simulink subsystem "DCDC_Converters_GenBat"  (R2024a)
settings: Solver=VariableStepAuto  StartTime=0.0  StopTime=10.0  RelTol=1e-3
undefined symbols (not defined in the file): C_bus, DCDC, L_boost, R_boost, rPre
settings Model: Creator=Henrique Mesquita  LastModifiedBy=henri

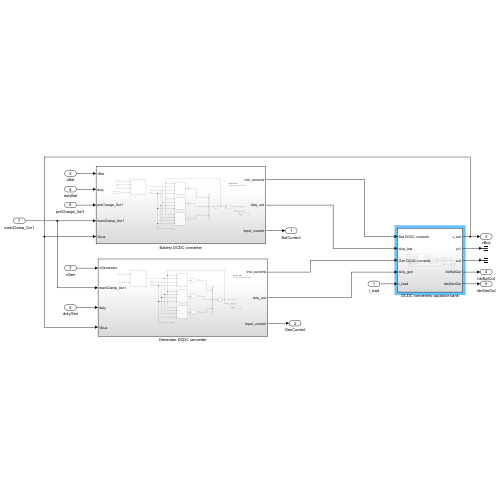
[thumbnail: Simulink's stored preview of the top-level diagram]
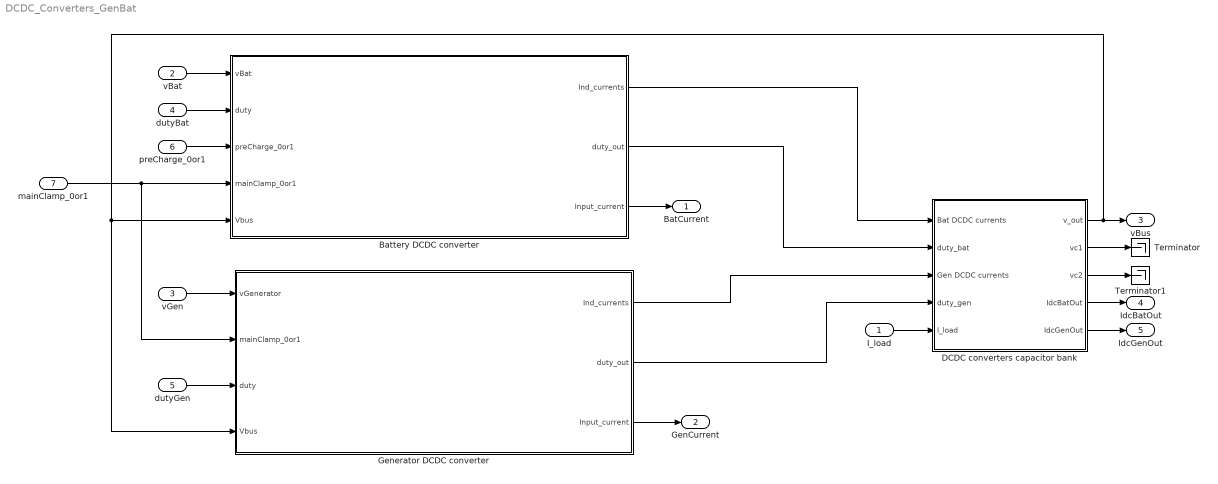
== system DCDC_Converters_GenBat ==
  I_load : Inport
  vBat : Inport  Port=2
  vGen : Inport  Port=3
  dutyBat : Inport  Port=4
  dutyGen : Inport  Port=5
  preCharge_0or1 : Inport  Port=6  OutDataTypeStr=int8
  mainClamp_0or1 : Inport  Port=7  OutDataTypeStr=int8
  Battery DCDC converter : Subsystem
  DCDC converters capacitor bank : Subsystem
  Generator DCDC converter : Subsystem
  Terminator : Terminator
  Terminator1 : Terminator
  BatCurrent : Outport
  GenCurrent : Outport  Port=2
  vBus : Outport  Port=3
  IdcBatOut : Outport  Port=4
  IdcGenOut : Outport  Port=5
  wires:
  Battery DCDC converter/1(Ind_currents) -> DCDC converters capacitor bank/1(Bat DCDC currents)
  Generator DCDC converter/1(Ind_currents) -> DCDC converters capacitor bank/3(Gen DCDC currents)
  Battery DCDC converter/2(duty_out) -> DCDC converters capacitor bank/2(duty_bat)
  Generator DCDC converter/2(duty_out) -> DCDC converters capacitor bank/4(duty_gen)
  I_load/1 -> DCDC converters capacitor bank/5(I_load)
  Battery DCDC converter/3(Input_current) -> BatCurrent/1
  Generator DCDC converter/3(Input_current) -> GenCurrent/1
  vGen/1 -> Generator DCDC converter/1(vGenerator)
  dutyGen/1 -> Generator DCDC converter/3(duty)
  preCharge_0or1/1 -> Battery DCDC converter/3(preCharge_0or1)
  mainClamp_0or1/1 -> Generator DCDC converter/2(mainClamp_0or1), Battery DCDC converter/4(mainClamp_0or1)
  dutyBat/1 -> Battery DCDC converter/2(duty)
  vBat/1 -> Battery DCDC converter/1(vBat)
  DCDC converters capacitor bank/1(v_out) -> vBus/1, Generator DCDC converter/4(Vbus), Battery DCDC converter/5(Vbus)
  DCDC converters capacitor bank/2(vc1) -> Terminator/1
  DCDC converters capacitor bank/3(vc2) -> Terminator1/1
  DCDC converters capacitor bank/4(IdcBatOut) -> IdcBatOut/1
  DCDC converters capacitor bank/5(IdcGenOut) -> IdcGenOut/1

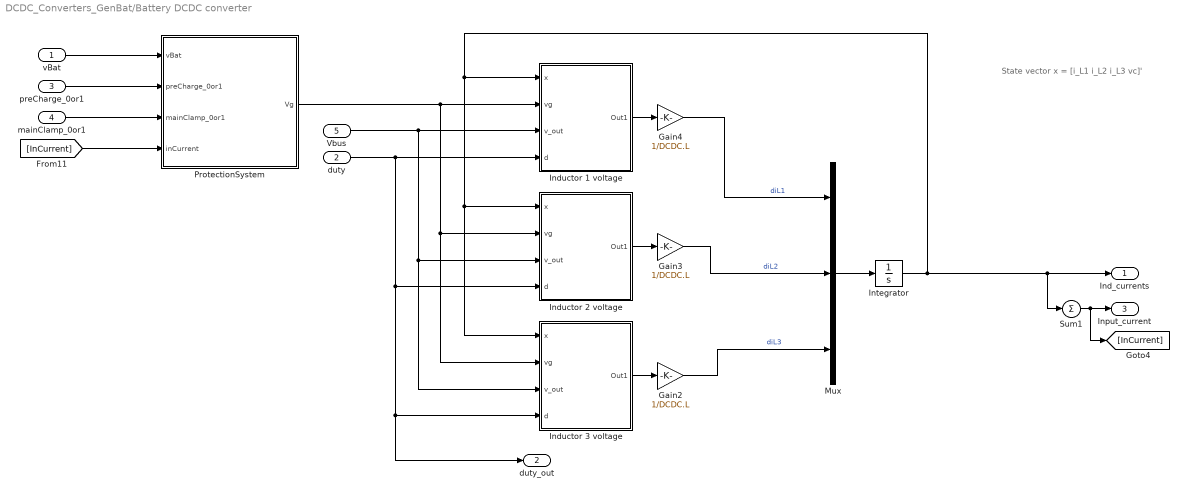
== system DCDC_Converters_GenBat/Battery DCDC converter ==
  note: State vector
      | x = [i_L1 i_L2 i_L3 vc]'
  vBat : Inport
  duty : Inport  Port=2
  preCharge_0or1 : Inport  Port=3
  mainClamp_0or1 : Inport  Port=4
  Vbus : Inport  Port=5
  Gain2 : Gain  Gain=1/DCDC.L
  Gain3 : Gain  Gain=1/DCDC.L
  Gain4 : Gain  Gain=1/DCDC.L
  Inductor 1 voltage : Subsystem
  Inductor 2 voltage : Subsystem
  Inductor 3 voltage : Subsystem
  Integrator : Integrator  InitialCondition=[0;0;0]
  Mux : Mux  Inputs=3
  ProtectionSystem : Subsystem
  Sum1 : Sum  Inputs=+
  Ind_currents : Outport
  duty_out : Outport  Port=2
  Input_current : Outport  Port=3
  wires:
  [InCurrent] -> ProtectionSystem/4(inCurrent)
  mainClamp_0or1/1 -> ProtectionSystem/3(mainClamp_0or1)
  preCharge_0or1/1 -> ProtectionSystem/2(preCharge_0or1)
  vBat/1 -> ProtectionSystem/1(vBat)
  Sum1/1 -> Input_current/1, [InCurrent]
  duty/1 -> duty_out/1, Inductor 3 voltage/4(d), Inductor 2 voltage/4(d), Inductor 1 voltage/4(d)
  ProtectionSystem/1(Vg) -> Inductor 2 voltage/2(vg), Inductor 3 voltage/2(vg), Inductor 1 voltage/2(vg)
  Vbus/1 -> Inductor 1 voltage/3(v_out), Inductor 3 voltage/3(v_out), Inductor 2 voltage/3(v_out)
  Integrator/1 -> Inductor 1 voltage/1(x), Inductor 3 voltage/1(x), Inductor 2 voltage/1(x), Ind_currents/1, Sum1/1
  Gain4/1 -> Mux/1  "diL1"
  Gain3/1 -> Mux/2  "diL2"
  Gain2/1 -> Mux/3  "diL3"
  Inductor 1 voltage/1(Out1) -> Gain4/1
  Inductor 3 voltage/1(Out1) -> Gain2/1
  Inductor 2 voltage/1(Out1) -> Gain3/1
  Mux/1 -> Integrator/1

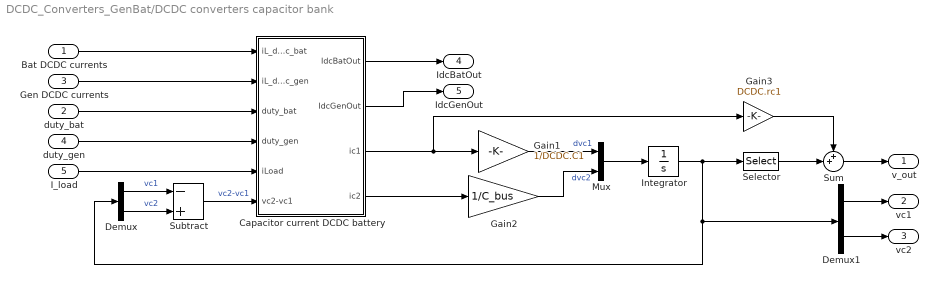
== system DCDC_Converters_GenBat/DCDC converters capacitor bank ==
  Bat DCDC currents : Inport
  duty_bat : Inport  Port=2
  Gen DCDC currents : Inport  Port=3
  duty_gen : Inport  Port=4
  I_load : Inport  Port=5
  Capacitor current DCDC battery : Subsystem
  Demux : Demux  Outputs=2
  Demux1 : Demux  Outputs=2
  Gain1 : Gain  Gain=1/DCDC.C1
  Gain2 : Gain  Gain=1/C_bus
  Gain3 : Gain  Gain=DCDC.rc1
  Integrator : Integrator
  Mux : Mux  Inputs=2
  Selector : Selector  InputPortWidth=2  IndexOptions=Index vector (dialog)  Indices=[1]  OutputSizes=1
  Subtract : Sum  Inputs=-+
  Sum : Sum  Inputs=++|
  v_out : Outport
  vc1 : Outport  Port=2
  vc2 : Outport  Port=3
  IdcBatOut : Outport  Port=4
  IdcGenOut : Outport  Port=5
  wires:
  Mux/1 -> Integrator/1
  Demux/1 -> Subtract/1  "vc1"
  Demux/2 -> Subtract/2  "vc2"
  Bat DCDC currents/1 -> Capacitor current DCDC battery/1(iL_dcdc_bat)
  Gen DCDC currents/1 -> Capacitor current DCDC battery/2(iL_dcdc_gen)
  I_load/1 -> Capacitor current DCDC battery/5(iLoad)
  Subtract/1 -> Capacitor current DCDC battery/6(vc2-vc1)  "vc2-vc1"
  Capacitor current DCDC battery/4(ic2) -> Gain2/1
  Capacitor current DCDC battery/3(ic1) -> Gain3/1, Gain1/1
  Gain1/1 -> Mux/1  "dvc1"
  Gain2/1 -> Mux/2  "dvc2"
  duty_bat/1 -> Capacitor current DCDC battery/3(duty_bat)
  duty_gen/1 -> Capacitor current DCDC battery/4(duty_gen)
  Integrator/1 -> Selector/1, Demux1/1, Demux/1
  Gain3/1 -> Sum/1
  Selector/1 -> Sum/2
  Sum/1 -> v_out/1
  Demux1/1 -> vc1/1
  Demux1/2 -> vc2/1
  Capacitor current DCDC battery/1(IdcBatOut) -> IdcBatOut/1
  Capacitor current DCDC battery/2(IdcGenOut) -> IdcGenOut/1

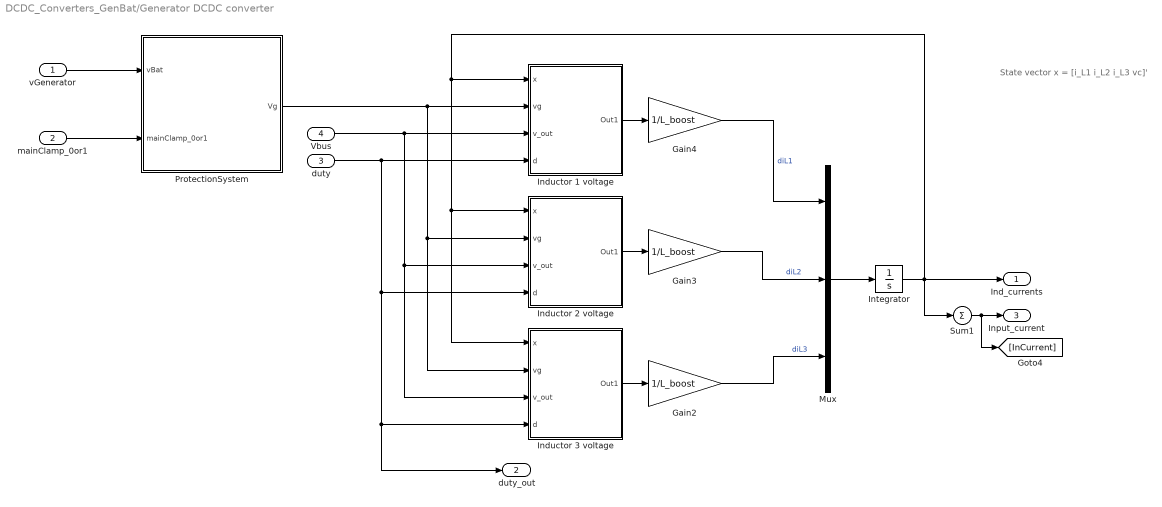
== system DCDC_Converters_GenBat/Generator DCDC converter ==
  note: State vector
      | x = [i_L1 i_L2 i_L3 vc]'
  vGenerator : Inport
  mainClamp_0or1 : Inport  Port=2
  duty : Inport  Port=3
  Vbus : Inport  Port=4
  Gain2 : Gain  Gain=1/L_boost
  Gain3 : Gain  Gain=1/L_boost
  Gain4 : Gain  Gain=1/L_boost
  Inductor 1 voltage : Subsystem
  Inductor 2 voltage : Subsystem
  Inductor 3 voltage : Subsystem
  Integrator : Integrator  InitialCondition=[0;0;0]  LimitOutput=on  LowerSaturationLimit=0
  Mux : Mux  Inputs=3
  ProtectionSystem : Subsystem
  Sum1 : Sum  Inputs=+
  Ind_currents : Outport
  duty_out : Outport  Port=2
  Input_current : Outport  Port=3
  wires:
  mainClamp_0or1/1 -> ProtectionSystem/2(mainClamp_0or1)
  vGenerator/1 -> ProtectionSystem/1(vBat)
  ProtectionSystem/1(Vg) -> Inductor 3 voltage/2(vg), Inductor 2 voltage/2(vg), Inductor 1 voltage/2(vg)
  Vbus/1 -> Inductor 1 voltage/3(v_out), Inductor 3 voltage/3(v_out), Inductor 2 voltage/3(v_out)
  duty/1 -> Inductor 2 voltage/4(d), Inductor 3 voltage/4(d), duty_out/1, Inductor 1 voltage/4(d)
  Integrator/1 -> Ind_currents/1, Sum1/1, Inductor 1 voltage/1(x), Inductor 3 voltage/1(x), Inductor 2 voltage/1(x)
  Inductor 3 voltage/1(Out1) -> Gain2/1
  Gain3/1 -> Mux/2  "diL2"
  Inductor 2 voltage/1(Out1) -> Gain3/1
  Inductor 1 voltage/1(Out1) -> Gain4/1
  Sum1/1 -> Input_current/1, [InCurrent]
  Gain4/1 -> Mux/1  "diL1"
  Mux/1 -> Integrator/1
  Gain2/1 -> Mux/3  "diL3"

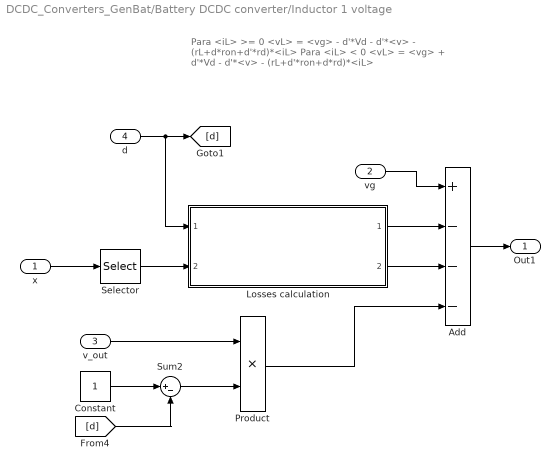
== system DCDC_Converters_GenBat/Battery DCDC converter/Inductor 1 voltage ==
  note: Para <iL> >= 0
      | <vL> = <vg> - d'*Vd - d'*<v> - (rL+d*ron+d'*rd)*<iL>
      | Para <iL> < 0
      | <vL> = <vg> + d'*Vd - d'*<v> - (rL+d'*ron+d*rd)*<iL>
  x : Inport
  vg : Inport  Port=2
  v_out : Inport  Port=3
  d : Inport  Port=4
  Add : Sum  Inputs=+---
  Constant : Constant
  Losses calculation : Subsystem  ReferencedSubsystem=Losses_calculation
  Product : Product
  Selector : Selector  InputPortWidth=3  IndexOptions=Index vector (dialog)  Indices=[1]  OutputSizes=1
  Sum2 : Sum  Inputs=|+-
  Out1 : Outport
  wires:
  Losses calculation/2 -> Add/3
  Losses calculation/1 -> Add/2
  [d] -> Sum2/2
  Sum2/1 -> Product/2
  Constant/1 -> Sum2/1
  Add/1 -> Out1/1
  Selector/1 -> Losses calculation/2
  v_out/1 -> Product/1
  d/1 -> [d], Losses calculation/1
  x/1 -> Selector/1
  Product/1 -> Add/4
  vg/1 -> Add/1

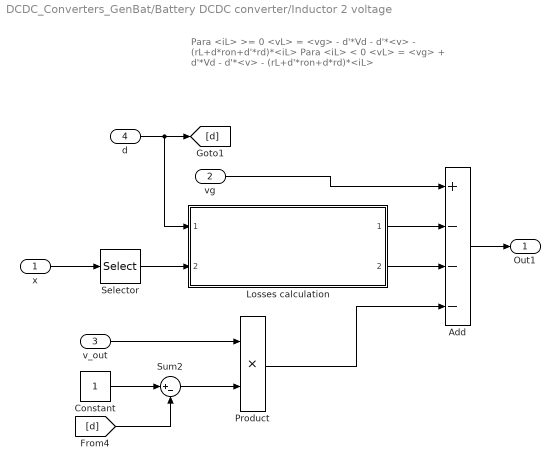
== system DCDC_Converters_GenBat/Battery DCDC converter/Inductor 2 voltage ==
  note: Para <iL> >= 0
      | <vL> = <vg> - d'*Vd - d'*<v> - (rL+d*ron+d'*rd)*<iL>
      | Para <iL> < 0
      | <vL> = <vg> + d'*Vd - d'*<v> - (rL+d'*ron+d*rd)*<iL>
  x : Inport
  vg : Inport  Port=2
  v_out : Inport  Port=3
  d : Inport  Port=4
  Add : Sum  Inputs=+---
  Constant : Constant
  Losses calculation : Subsystem  ReferencedSubsystem=Losses_calculation
  Product : Product
  Selector : Selector  InputPortWidth=3  IndexOptions=Index vector (dialog)  Indices=[2]  OutputSizes=1
  Sum2 : Sum  Inputs=|+-
  Out1 : Outport
  wires:
  Losses calculation/2 -> Add/3
  Losses calculation/1 -> Add/2
  [d] -> Sum2/2
  Sum2/1 -> Product/2
  Constant/1 -> Sum2/1
  Add/1 -> Out1/1
  Selector/1 -> Losses calculation/2
  v_out/1 -> Product/1
  d/1 -> [d], Losses calculation/1
  x/1 -> Selector/1
  Product/1 -> Add/4
  vg/1 -> Add/1

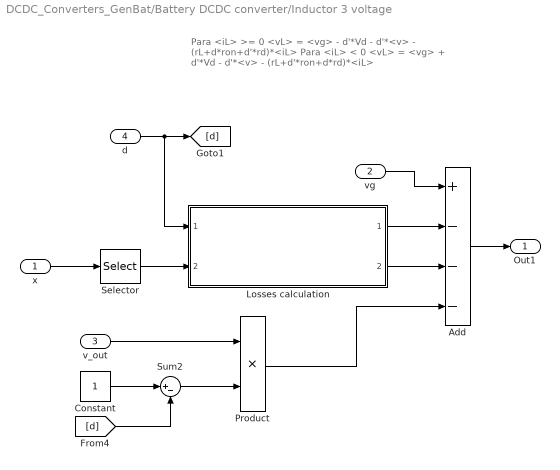
== system DCDC_Converters_GenBat/Battery DCDC converter/Inductor 3 voltage ==
  note: Para <iL> >= 0
      | <vL> = <vg> - d'*Vd - d'*<v> - (rL+d*ron+d'*rd)*<iL>
      | Para <iL> < 0
      | <vL> = <vg> + d'*Vd - d'*<v> - (rL+d'*ron+d*rd)*<iL>
  x : Inport
  vg : Inport  Port=2
  v_out : Inport  Port=3
  d : Inport  Port=4
  Add : Sum  Inputs=+---
  Constant : Constant
  Losses calculation : Subsystem  ReferencedSubsystem=Losses_calculation
  Product : Product
  Selector : Selector  InputPortWidth=3  IndexOptions=Index vector (dialog)  Indices=[3]  OutputSizes=1
  Sum2 : Sum  Inputs=|+-
  Out1 : Outport
  wires:
  Losses calculation/2 -> Add/3
  Losses calculation/1 -> Add/2
  [d] -> Sum2/2
  Sum2/1 -> Product/2
  Constant/1 -> Sum2/1
  Add/1 -> Out1/1
  Selector/1 -> Losses calculation/2
  v_out/1 -> Product/1
  d/1 -> [d], Losses calculation/1
  x/1 -> Selector/1
  Product/1 -> Add/4
  vg/1 -> Add/1

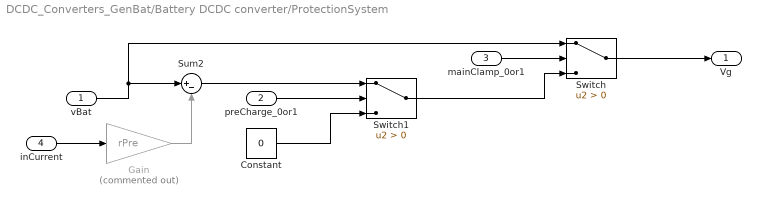
== system DCDC_Converters_GenBat/Battery DCDC converter/ProtectionSystem ==
  vBat : Inport
  preCharge_0or1 : Inport  Port=2
  mainClamp_0or1 : Inport  Port=3
  inCurrent : Inport  Port=4
  Constant : Constant  Value=0
  Gain : Gain  Commented=on  Gain=rPre
  Sum2 : Sum  Inputs=|+-
  Switch : Switch  Criteria=u2 > Threshold  SaturateOnIntegerOverflow=off  InputSameDT=off
  Switch1 : Switch  Criteria=u2 > Threshold  SaturateOnIntegerOverflow=off  InputSameDT=off
  Vg : Outport
  wires:
  Sum2/1 -> Switch1/1
  Switch1/1 -> Switch/3
  Constant/1 -> Switch1/3
  Switch/1 -> Vg/1
  vBat/1 -> Sum2/1, Switch/1
  mainClamp_0or1/1 -> Switch/2
  Gain/1 -> Sum2/2
  preCharge_0or1/1 -> Switch1/2
  inCurrent/1 -> Gain/1

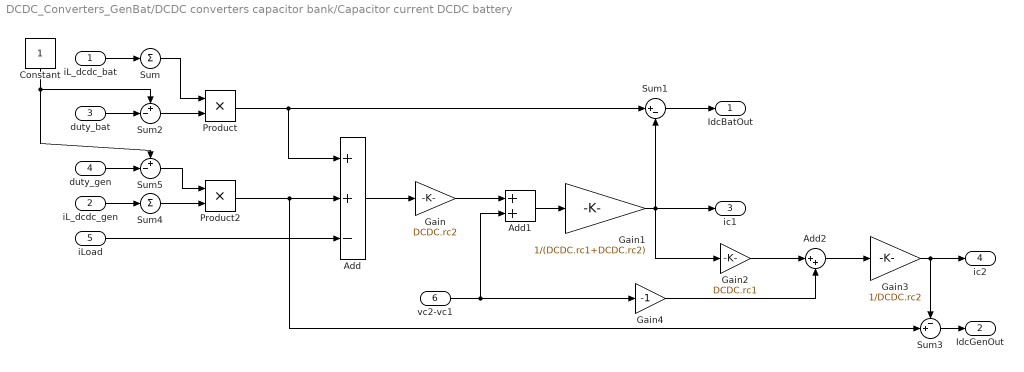
== system DCDC_Converters_GenBat/DCDC converters capacitor bank/Capacitor current DCDC battery ==
  iL_dcdc_bat : Inport
  iL_dcdc_gen : Inport  Port=2
  duty_bat : Inport  Port=3
  duty_gen : Inport  Port=4
  iLoad : Inport  Port=5
  vc2-vc1 : Inport  Port=6
  Add : Sum  Inputs=++-
  Add1 : Sum
  Add2 : Sum  Inputs=|++
  Constant : Constant
  Gain : Gain  Gain=DCDC.rc2
  Gain1 : Gain  Gain=1/(DCDC.rc1+DCDC.rc2)
  Gain2 : Gain  Gain=DCDC.rc1
  Gain3 : Gain  Gain=1/DCDC.rc2
  Gain4 : Gain  Gain=-1
  Product : Product
  Product2 : Product
  Sum : Sum  Inputs=+
  Sum1 : Sum  Inputs=|+-
  Sum2 : Sum  Inputs=+-|
  Sum3 : Sum  Inputs=-+|
  Sum4 : Sum  Inputs=+
  Sum5 : Sum  Inputs=+-|
  IdcBatOut : Outport
  IdcGenOut : Outport  Port=2
  ic1 : Outport  Port=3
  ic2 : Outport  Port=4
  wires:
  iL_dcdc_bat/1 -> Sum/1
  Add1/1 -> Gain1/1
  Gain/1 -> Add1/1
  Add/1 -> Gain/1
  iLoad/1 -> Add/3
  Sum/1 -> Product/1
  Product2/1 -> Sum3/2, Add/2
  Sum2/1 -> Product/2
  duty_bat/1 -> Sum2/2
  iL_dcdc_gen/1 -> Sum4/1
  duty_gen/1 -> Sum5/2
  Constant/1 -> Sum5/1, Sum2/1
  Sum5/1 -> Product2/1
  Sum4/1 -> Product2/2
  Product/1 -> Add/1, Sum1/1
  Sum1/1 -> IdcBatOut/1
  Gain3/1 -> Sum3/1, ic2/1
  vc2-vc1/1 -> Add1/2, Gain4/1
  Gain2/1 -> Add2/1
  Gain1/1 -> Gain2/1, ic1/1, Sum1/2
  Add2/1 -> Gain3/1
  Gain4/1 -> Add2/2
  Sum3/1 -> IdcGenOut/1

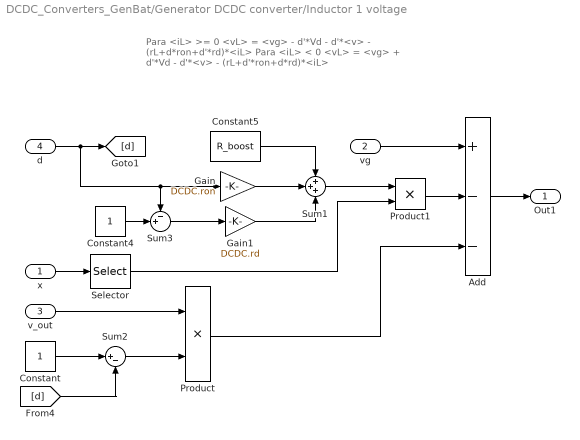
== system DCDC_Converters_GenBat/Generator DCDC converter/Inductor 1 voltage ==
  note: Para <iL> >= 0
      | <vL> = <vg> - d'*Vd - d'*<v> - (rL+d*ron+d'*rd)*<iL>
      | Para <iL> < 0
      | <vL> = <vg> + d'*Vd - d'*<v> - (rL+d'*ron+d*rd)*<iL>
  x : Inport
  vg : Inport  Port=2
  v_out : Inport  Port=3
  d : Inport  Port=4
  Add : Sum  Inputs=+--
  Constant : Constant
  Constant4 : Constant
  Constant5 : Constant  Value=R_boost
  Gain : Gain  Gain=DCDC.ron
  Gain1 : Gain  Gain=DCDC.rd
  Product : Product
  Product1 : Product
  Selector : Selector  InputPortWidth=3  IndexOptions=Index vector (dialog)  Indices=[1]  OutputSizes=1
  Sum1 : Sum  Inputs=+++
  Sum2 : Sum  Inputs=|+-
  Sum3 : Sum  Inputs=-+|
  Out1 : Outport
  wires:
  Product1/1 -> Add/2
  [d] -> Sum2/2
  Sum2/1 -> Product/2
  Constant/1 -> Sum2/1
  Add/1 -> Out1/1
  v_out/1 -> Product/1
  x/1 -> Selector/1
  Product/1 -> Add/3
  vg/1 -> Add/1
  Sum1/1 -> Product1/1
  Sum3/1 -> Gain1/1
  d/1 -> Gain/1, Sum3/1, [d]
  Gain1/1 -> Sum1/3
  Gain/1 -> Sum1/2
  Constant4/1 -> Sum3/2
  Selector/1 -> Product1/2
  Constant5/1 -> Sum1/1

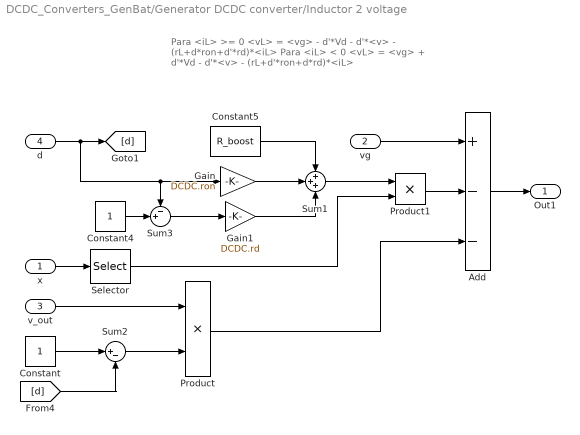
== system DCDC_Converters_GenBat/Generator DCDC converter/Inductor 2 voltage ==
  note: Para <iL> >= 0
      | <vL> = <vg> - d'*Vd - d'*<v> - (rL+d*ron+d'*rd)*<iL>
      | Para <iL> < 0
      | <vL> = <vg> + d'*Vd - d'*<v> - (rL+d'*ron+d*rd)*<iL>
  x : Inport
  vg : Inport  Port=2
  v_out : Inport  Port=3
  d : Inport  Port=4
  Add : Sum  Inputs=+--
  Constant : Constant
  Constant4 : Constant
  Constant5 : Constant  Value=R_boost
  Gain : Gain  Gain=DCDC.ron
  Gain1 : Gain  Gain=DCDC.rd
  Product : Product
  Product1 : Product
  Selector : Selector  InputPortWidth=3  IndexOptions=Index vector (dialog)  Indices=[2]  OutputSizes=1
  Sum1 : Sum  Inputs=+++
  Sum2 : Sum  Inputs=|+-
  Sum3 : Sum  Inputs=-+|
  Out1 : Outport
  wires:
  Add/1 -> Out1/1
  Selector/1 -> Product1/2
  d/1 -> Gain/1, Sum3/1, [d]
  Constant/1 -> Sum2/1
  Product1/1 -> Add/2
  Constant4/1 -> Sum3/2
  Constant5/1 -> Sum1/1
  Gain1/1 -> Sum1/3
  Gain/1 -> Sum1/2
  v_out/1 -> Product/1
  Sum3/1 -> Gain1/1
  vg/1 -> Add/1
  [d] -> Sum2/2
  Product/1 -> Add/3
  Sum2/1 -> Product/2
  x/1 -> Selector/1
  Sum1/1 -> Product1/1

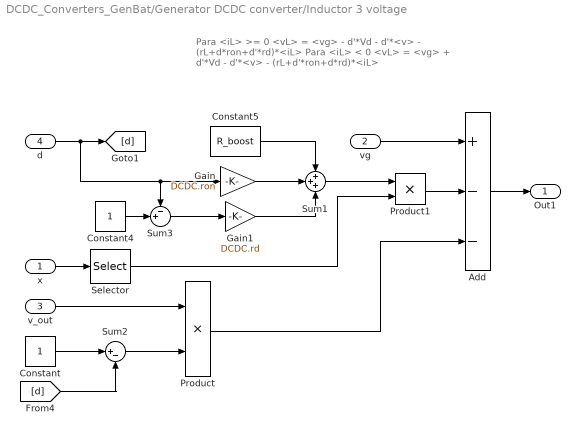
== system DCDC_Converters_GenBat/Generator DCDC converter/Inductor 3 voltage ==
  note: Para <iL> >= 0
      | <vL> = <vg> - d'*Vd - d'*<v> - (rL+d*ron+d'*rd)*<iL>
      | Para <iL> < 0
      | <vL> = <vg> + d'*Vd - d'*<v> - (rL+d'*ron+d*rd)*<iL>
  x : Inport
  vg : Inport  Port=2
  v_out : Inport  Port=3
  d : Inport  Port=4
  Add : Sum  Inputs=+--
  Constant : Constant
  Constant4 : Constant
  Constant5 : Constant  Value=R_boost
  Gain : Gain  Gain=DCDC.ron
  Gain1 : Gain  Gain=DCDC.rd
  Product : Product
  Product1 : Product
  Selector : Selector  InputPortWidth=3  IndexOptions=Index vector (dialog)  Indices=[1]  OutputSizes=1
  Sum1 : Sum  Inputs=+++
  Sum2 : Sum  Inputs=|+-
  Sum3 : Sum  Inputs=-+|
  Out1 : Outport
  wires:
  Add/1 -> Out1/1
  Selector/1 -> Product1/2
  d/1 -> Gain/1, Sum3/1, [d]
  Constant/1 -> Sum2/1
  Product1/1 -> Add/2
  Constant4/1 -> Sum3/2
  Constant5/1 -> Sum1/1
  Gain1/1 -> Sum1/3
  Gain/1 -> Sum1/2
  v_out/1 -> Product/1
  Sum3/1 -> Gain1/1
  vg/1 -> Add/1
  [d] -> Sum2/2
  Product/1 -> Add/3
  Sum2/1 -> Product/2
  x/1 -> Selector/1
  Sum1/1 -> Product1/1

== system DCDC_Converters_GenBat/Generator DCDC converter/ProtectionSystem ==
  vBat : Inport
  mainClamp_0or1 : Inport  Port=2
  Constant : Constant  Value=0
  Switch : Switch  Criteria=u2 > Threshold  SaturateOnIntegerOverflow=off  InputSameDT=off
  Vg : Outport
  wires:
  Constant/1 -> Switch/3
  Switch/1 -> Vg/1
  vBat/1 -> Switch/1
  mainClamp_0or1/1 -> Switch/2
